simulink model "dynamik_3"  (R2016b)
settings: Solver=ode45  StartTime=0.0  StopTime=80  RelTol=1e-3
values from neighbouring files (symbols this model uses):
  A = 0.05    [Test_m1_init.m]
  a_acc = 1    [Test_m1_init.m]    (also in Test_m2_init.m = 5.5)
  a_de = 1    [Test_m1_init.m]    (also in Test_m2_init.m = 5.5)
  d_2 = 0.15    [Test_m1_init.m]
  dot_phi_soll = 1    [Test_m2_init.m]
  I_R = Mass*(0.5*L)^2    (= 0.08)    [Test_m1_init.m]    (also in Test_m2_init.m)
  L = 0.4    [Test_m1_init.m]    (also in Test_m2_init.m)
  l = 0.2    [Test_m1_init.m]    (also in Test_m2_init.m)
  m = 0.5    [Test_m1_init.m]    (also in Test_m2_init.m)
  Mass = 2    [Test_m1_init.m]    (also in Test_m2_init.m)
libraries: simulink x2
settings Model: Creator=Alexa  LastModifiedBy=Alexa

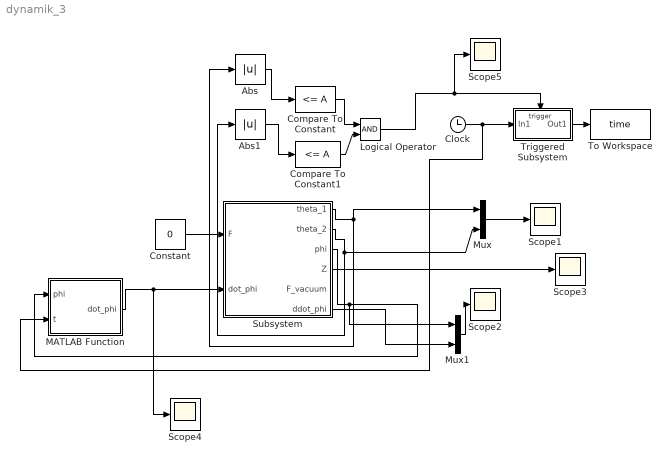
== system dynamik_3 ==
  Abs : Abs
  Abs1 : Abs
  Clock : Clock
  Compare To Constant : simulink/Logic and Bit Operations/Compare To Constant  relop=<=  const=A  OutDataTypeStr=boolean
  Compare To Constant1 : simulink/Logic and Bit Operations/Compare To Constant  relop=<=  const=A  OutDataTypeStr=boolean
  Constant : Constant  Value=0
  Logical Operator : Logic  AllPortsSameDT=off  OutDataTypeStr=boolean
  MATLAB Function : MATLAB Function  TreatAsAtomicUnit=on
  Mux : Mux  Inputs=2
  Mux1 : Mux  Inputs=2
  Scope{1..5} (5 alike) : Scope
  Subsystem : Subsystem
  To Workspace : ToWorkspace  VariableName=time  SaveFormat=Timeseries  SampleTime=-1
  Triggered Subsystem : Subsystem  TreatAsAtomicUnit=on
  wires:
  Subsystem/2(theta_2) -> Abs1/1, Mux/2
  Subsystem/1(theta_1) -> Abs/1, Mux/1
  Constant/1 -> Subsystem/1(F)
  Subsystem/3(phi) -> MATLAB Function/1(phi), Mux1/1
  Subsystem/4(Z) -> Scope3/1
  Compare To Constant/1 -> Logical Operator/1
  Compare To Constant1/1 -> Logical Operator/2
  Logical Operator/1 -> Scope5/1, Triggered Subsystem/Trigger
  Triggered Subsystem/1(Out1) -> To Workspace/1
  MATLAB Function/1(dot_phi) -> Subsystem/2(dot_phi), Scope4/1
  Subsystem/6(ddot_phi) -> Mux1/2
  Mux1/1 -> Scope2/1
  Clock/1 -> MATLAB Function/2(t), Triggered Subsystem/1(In1)
  Mux/1 -> Scope1/1
  Abs/1 -> Compare To Constant/1
  Abs1/1 -> Compare To Constant1/1

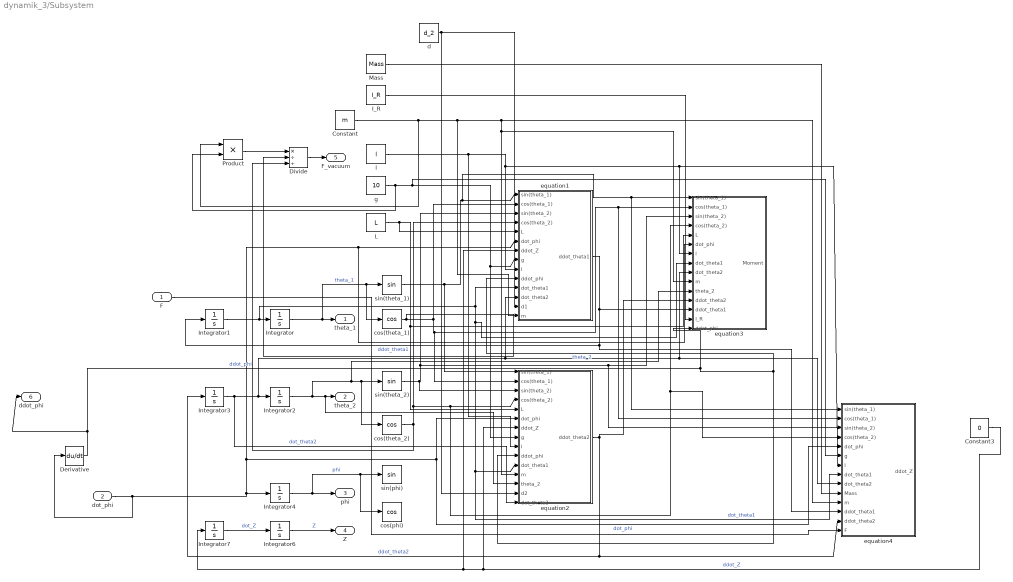
== system dynamik_3/Subsystem ==
  F : Inport
  dot_phi : Inport  Port=2
  Constant : Constant  Value=m
  Constant3 : Constant  Value=0
  Derivative : Derivative
  Divide : Product  Inputs=*//
  I_R : Constant  Value=I_R
  Integrator{,1..4,6..7} (7 alike) : Integrator
  L : Constant  Value=L
  Mass : Constant  Value=Mass
  Product : Product
  cos(phi) : Trigonometry  Operator=cos
  cos(theta_1) : Trigonometry  Operator=cos
  cos(theta_2) : Trigonometry  Operator=cos
  d : Constant  Value=d_2
  equation1 : Subsystem
  equation2 : Subsystem
  equation3 : Subsystem
  equation4 : Subsystem
  g : Constant  Value=10
  l : Constant  Value=l
  sin(phi) : Trigonometry
  sin(theta_1) : Trigonometry
  sin(theta_2) : Trigonometry
  theta_1 : Outport
  theta_2 : Outport  Port=2
  phi : Outport  Port=3
  Z : Outport  Port=4
  F_vacuum : Outport  Port=5
  ddot_phi : Outport  Port=6
  wires:
  Integrator/1 -> cos(theta_1)/1, sin(theta_1)/1, theta_1/1  "theta_1"
  Integrator1/1 -> equation1/11(dot_theta1), equation3/8(dot_theta1), equation4/8(dot_theta1), equation2/11(dot_theta1), Integrator/1  "dot_theta1"
  Integrator2/1 -> equation3/11(theta_2), cos(theta_2)/1, sin(theta_2)/1, equation2/13(theta_2), theta_2/1  "theta_2"
  Integrator3/1 -> equation2/15(dot_theta2), equation4/9(dot_theta2), equation3/9(dot_theta2), equation1/12(dot_theta2), Integrator2/1  "dot_theta2"
  Integrator4/1 -> cos(phi)/1, sin(phi)/1, phi/1  "phi"
  Integrator6/1 -> Z/1  "Z"
  Integrator7/1 -> Integrator6/1  "dot_Z"
  equation1/1(ddot_theta1) -> equation3/13(ddot_theta1), equation4/12(ddot_theta1), Integrator1/1  "ddot_theta1"
  equation2/1(ddot_theta2) -> equation3/12(ddot_theta2), equation4/13(ddot_theta2), Integrator3/1  "ddot_theta2"
  Constant3/1 -> equation1/7(ddot_Z), Integrator7/1, equation2/7(ddot_Z)  "ddot_Z"
  sin(theta_1)/1 -> equation2/1(sin(theta_1)), equation4/1(sin(theta_1)), equation3/1(sin(theta_1)), equation1/1(sin(theta_1))
  cos(theta_1)/1 -> Divide/2, equation2/2(cos(theta_1)), equation4/2(cos(theta_1)), equation3/2(cos(theta_1)), equation1/2(cos(theta_1))
  sin(theta_2)/1 -> equation2/3(sin(theta_2)), equation4/3(sin(theta_2)), equation3/3(sin(theta_2)), equation1/3(sin(theta_2))
  cos(theta_2)/1 -> Divide/3, equation4/4(cos(theta_2)), equation3/4(cos(theta_2)), equation2/4(cos(theta_2)), equation1/4(cos(theta_2))
  L/1 -> equation2/5(L), equation3/5(L), equation1/5(L)
  g/1 -> Product/2, equation4/6(g), equation2/8(g), equation1/8(g)
  l/1 -> equation2/9(l), equation4/7(l), equation3/7(l), equation1/9(l)
  Constant/1 -> Product/1, equation1/14(m), equation4/11(m), equation2/12(m), equation3/10(m)
  I_R/1 -> equation3/14(I_R)
  Mass/1 -> equation4/10(Mass)
  Product/1 -> Divide/1
  Divide/1 -> F_vacuum/1
  d/1 -> equation1/13(d1), equation2/14(d2)
  F/1 -> equation4/14(F)
  Derivative/1 -> ddot_phi/1, equation3/15("ddot_phi "), equation1/10(ddot_phi), equation2/10(ddot_phi)  "ddot_phi"
  dot_phi/1 -> Derivative/1, equation2/6(dot_phi), equation4/5(dot_phi), equation3/6(dot_phi), equation1/6(dot_phi), Integrator4/1  "dot_phi"

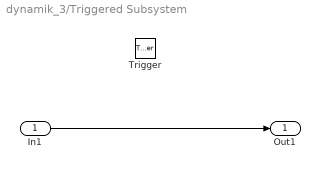
== system dynamik_3/Triggered Subsystem ==
  In1 : Inport
  Trigger : TriggerPort  VariantControl=Variant
  Out1 : Outport
  wires:
  In1/1 -> Out1/1

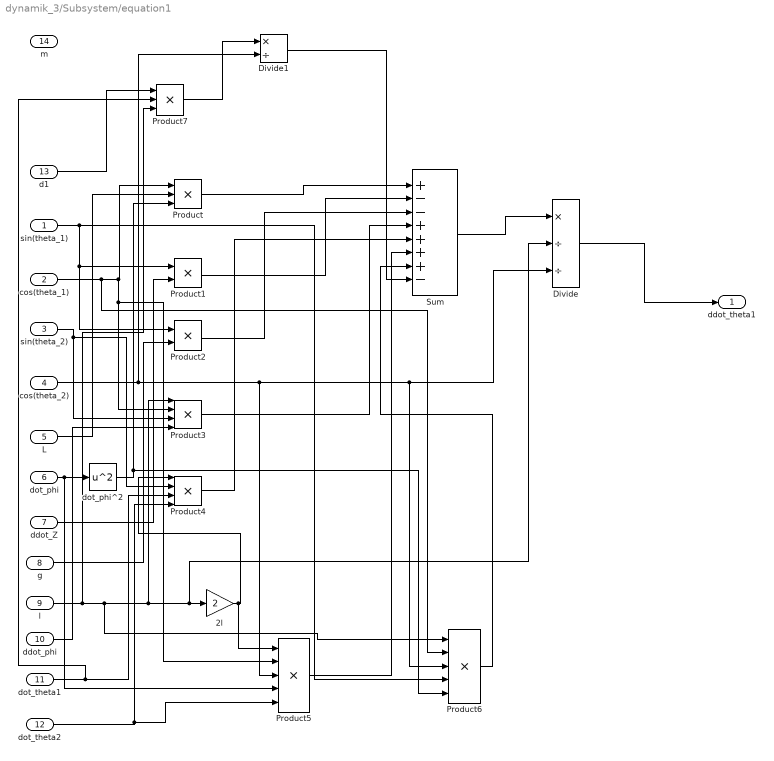
== system dynamik_3/Subsystem/equation1 ==
  sin(theta_1) : Inport
  cos(theta_1) : Inport  Port=2
  sin(theta_2) : Inport  Port=3
  cos(theta_2) : Inport  Port=4
  L : Inport  Port=5
  dot_phi : Inport  Port=6
  ddot_Z : Inport  Port=7
  g : Inport  Port=8
  l : Inport  Port=9
  ddot_phi : Inport  Port=10
  dot_theta1 : Inport  Port=11
  dot_theta2 : Inport  Port=12
  d1 : Inport  Port=13
  m : Inport  Port=14
  2l : Gain  Gain=2
  Divide : Product  Inputs=*//
  Divide1 : Product  Inputs=*/
  Product : Product  Inputs=3
  Product1 : Product
  Product2 : Product
  Product3 : Product  Inputs=4
  Product4 : Product  Inputs=4
  Product5 : Product  Inputs=5
  Product6 : Product  Inputs=5
  Product7 : Product  Inputs=3
  Sum : Sum  Inputs=+--++++-
  dot_phi^2 : Math  Operator=square  SaturateOnIntegerOverflow=on
  ddot_theta1 : Outport
  wires:
  dot_phi/1 -> Product5/4, dot_phi^2/1
  cos(theta_1)/1 -> Product6/2, Product5/2, Product3/2, Product/1
  L/1 -> Product/2
  dot_phi^2/1 -> Product6/5, Product/3
  Product/1 -> Sum/1
  sin(theta_1)/1 -> Product6/4, Product2/1, Product1/1
  Product1/1 -> Sum/2
  ddot_Z/1 -> Product1/2
  g/1 -> Product2/2
  Product2/1 -> Sum/3
  l/1 -> Product7/3, Product6/1, Divide/2, 2l/1, Product3/1
  sin(theta_2)/1 -> Product4/2, Product3/3
  Product3/1 -> Sum/4
  ddot_phi/1 -> Product3/4
  2l/1 -> Product5/1, Product4/1
  dot_theta1/1 -> Product7/2, Product4/3
  dot_theta2/1 -> Product5/5, Product4/4
  Product4/1 -> Sum/5
  cos(theta_2)/1 -> Divide1/2, Divide/3, Product6/3, Product5/3
  Product5/1 -> Sum/6
  Sum/1 -> Divide/1
  Product6/1 -> Sum/7
  Divide/1 -> ddot_theta1/1
  d1/1 -> Product7/1
  Product7/1 -> Divide1/1
  Divide1/1 -> Sum/8

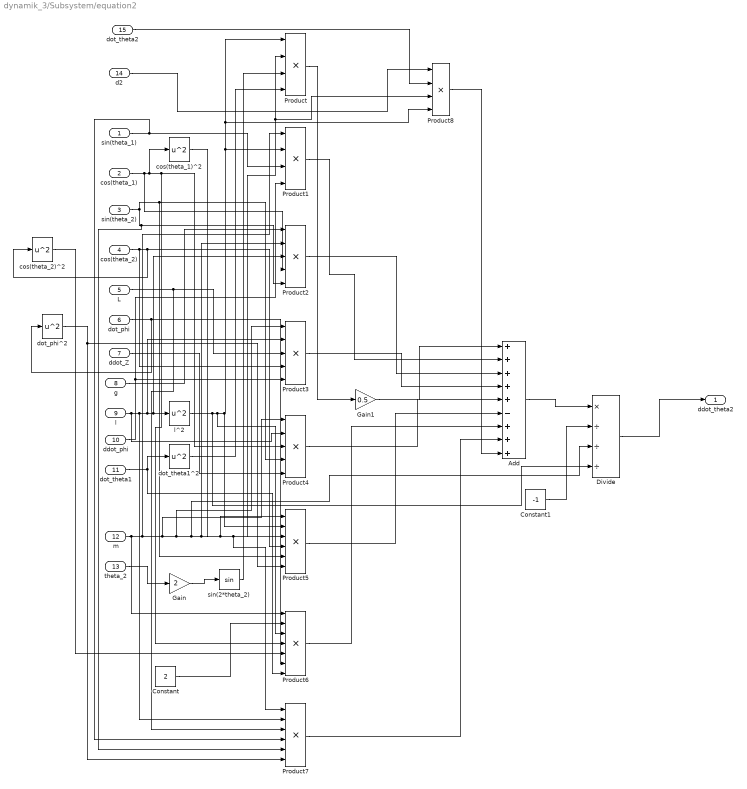
== system dynamik_3/Subsystem/equation2 ==
  sin(theta_1) : Inport
  cos(theta_1) : Inport  Port=2
  sin(theta_2) : Inport  Port=3
  cos(theta_2) : Inport  Port=4
  L : Inport  Port=5
  dot_phi : Inport  Port=6
  ddot_Z : Inport  Port=7
  g : Inport  Port=8
  l : Inport  Port=9
  ddot_phi : Inport  Port=10
  dot_theta1 : Inport  Port=11
  m : Inport  Port=12
  theta_2 : Inport  Port=13
  d2 : Inport  Port=14
  dot_theta2 : Inport  Port=15
  Add : Sum  Inputs=+++++-+++
  Constant : Constant  Value=2
  Constant1 : Constant  Value=-1
  Divide : Product  Inputs=*///
  Gain : Gain  Gain=2
  Gain1 : Gain  Gain=0.5
  Product : Product  Inputs=4
  Product1 : Product  Inputs=4
  Product2 : Product  Inputs=5
  Product3 : Product  Inputs=5
  Product4 : Product  Inputs=5
  Product5 : Product  Inputs=6
  Product6 : Product  Inputs=7
  Product7 : Product  Inputs=6
  Product8 : Product  Inputs=4
  cos(theta_1)^2 : Math  Operator=square  SaturateOnIntegerOverflow=on
  cos(theta_2)^2 : Math  Operator=square  SaturateOnIntegerOverflow=on
  dot_phi^2 : Math  Operator=square  SaturateOnIntegerOverflow=on
  dot_theta1^2 : Math  Operator=square  SaturateOnIntegerOverflow=on
  l^2 : Math  Operator=square  SaturateOnIntegerOverflow=on
  sin(2*theta_2) : Trigonometry
  ddot_theta2 : Outport
  wires:
  l/1 -> Product4/2, Product7/2, Product3/2, Product2/3, l^2/1
  l^2/1 -> Divide/4, Product6/3, Product5/2, Product8/4, Product/1, Product1/2
  m/1 -> Product6/1, Product1/1, Product4/1, Product3/1, Divide/3, Product2/2, Product5/1, Product8/3, Product/2
  theta_2/1 -> Gain/1
  Gain/1 -> sin(2*theta_2)/1
  sin(2*theta_2)/1 -> Product/3
  dot_theta1/1 -> Product6/7, dot_theta1^2/1
  dot_theta1^2/1 -> Product/4
  Product/1 -> Gain1/1
  Gain1/1 -> Add/1
  sin(theta_1)/1 -> Product7/4, Product1/3
  ddot_phi/1 -> Product1/4, Product3/5
  Product1/1 -> Add/2
  g/1 -> Product2/1
  cos(theta_1)/1 -> cos(theta_1)^2/1, Product6/4, Product4/3, Product2/4
  sin(theta_2)/1 -> Product7/5, Product2/5, Product5/5, Product4/4
  Product2/1 -> Add/3
  L/1 -> Product7/3, Product3/3
  cos(theta_2)/1 -> cos(theta_2)^2/1, Product5/4, Product3/4
  Product3/1 -> Add/4
  ddot_Z/1 -> Product4/5
  Product4/1 -> Add/5
  cos(theta_1)^2/1 -> Product7/1, Product5/3
  dot_phi/1 -> Product6/6, dot_phi^2/1
  dot_phi^2/1 -> Product7/6, Product5/6
  Product5/1 -> Add/6
  Constant/1 -> Product6/2
  cos(theta_2)^2/1 -> Product6/5
  Product6/1 -> Add/7
  Product7/1 -> Add/8
  Add/1 -> Divide/1
  Constant1/1 -> Divide/2
  Divide/1 -> ddot_theta2/1
  d2/1 -> Product8/1
  dot_theta2/1 -> Product8/2
  Product8/1 -> Add/9

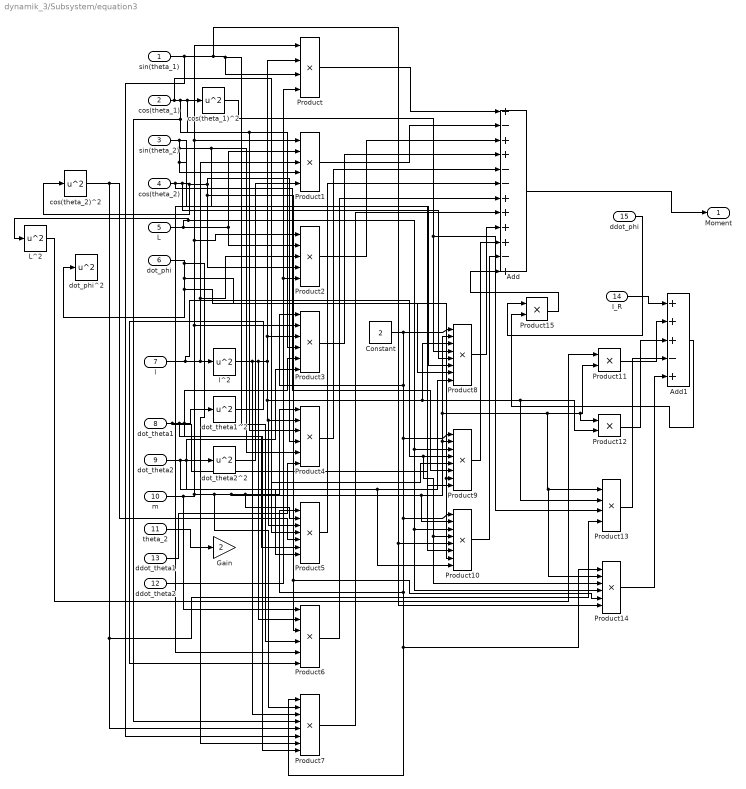
== system dynamik_3/Subsystem/equation3 ==
  sin(theta_1) : Inport
  cos(theta_1) : Inport  Port=2
  sin(theta_2) : Inport  Port=3
  cos(theta_2) : Inport  Port=4
  L : Inport  Port=5
  dot_phi : Inport  Port=6
  l : Inport  Port=7
  dot_theta1 : Inport  Port=8
  dot_theta2 : Inport  Port=9
  m : Inport  Port=10
  theta_2 : Inport  Port=11
  ddot_theta2 : Inport  Port=12
  ddot_theta1 : Inport  Port=13
  I_R : Inport  Port=14
  "ddot_phi " : Inport  Port=15
  Add : Sum  Inputs=+-++--++++-+
  Add1 : Sum  Inputs=+++-+
  Constant : Constant  Value=2
  Gain : Gain  Gain=2
  L^2 : Math  Operator=square  SaturateOnIntegerOverflow=on
  Product : Product  Inputs=4
  Product1 : Product  Inputs=5
  Product{7..10} (4 alike) : Product  Inputs=8
  Product11 : Product
  Product12 : Product
  Product13 : Product  Inputs=4
  Product{3..4,6,14} (4 alike) : Product  Inputs=6
  Product15 : Product
  Product2 : Product  Inputs=5
  Product5 : Product  Inputs=7
  cos(theta_1)^2 : Math  Operator=square  SaturateOnIntegerOverflow=on
  cos(theta_2)^2 : Math  Operator=square  SaturateOnIntegerOverflow=on
  dot_phi^2 : Math  Operator=square  SaturateOnIntegerOverflow=on
  dot_theta1^2 : Math  Operator=square  SaturateOnIntegerOverflow=on
  dot_theta2^2 : Math  Operator=square  SaturateOnIntegerOverflow=on
  l^2 : Math  Operator=square  SaturateOnIntegerOverflow=on
  "Moment " : Outport
  wires:
  l/1 -> Product14/3, Product10/4, Product9/4, Product2/3, Product1/3, l^2/1
  theta_2/1 -> Gain/1
  dot_theta1/1 -> Product9/8, Product7/8, Product5/6, Product3/5, dot_theta1^2/1
  cos(theta_1)/1 -> Product9/5, Product7/4, Product5/4, Product4/3, Product3/4, cos(theta_1)^2/1
  cos(theta_2)/1 -> Product9/6, Product8/5, Product4/4, Product14/5, Product6/3, Product2/4, cos(theta_2)^2/1
  dot_phi/1 -> Product7/7, Product8/7, Product10/7, Product9/7, dot_phi^2/1
  m/1 -> Product6/1, Product7/2, Product10/2, Product9/2, Product14/2, Product13/1, Product12/1, Product11/2, Product8/2, Product5/2, Product4/1, Product3/2, Product2/1, Product1/1, Product/1
  sin(theta_1)/1 -> Product7/6, Product14/6, Product10/5, Product6/4, Product/3
  ddot_theta2/1 -> Product2/5, Product/4
  Product/1 -> Add/1
  L/1 -> L^2/1, Product14/4, Product10/3, Product9/3, Product2/2, Product1/2
  sin(theta_2)/1 -> Product10/6, Product6/5, Product4/5, Product8/6, Product1/4
  dot_theta2^2/1 -> Product1/5
  Product1/1 -> Add/2
  Product2/1 -> Add/3
  Constant/1 -> Product8/1, Product9/1, Product10/1, Product14/1, Product7/1, Product5/1, Product3/1
  Product3/1 -> Add/4
  ddot_theta1/1 -> Product4/6
  Product4/1 -> Add/5
  cos(theta_2)^2/1 -> Product13/4, Product7/5, Product5/5
  Product5/1 -> Add/6
  dot_theta1^2/1 -> Product6/6
  Product6/1 -> Add/7
  Product7/1 -> Add/8
  cos(theta_1)^2/1 -> Product13/3, Product8/4
  Product8/1 -> Add/9
  Product9/1 -> Add/10
  dot_theta2/1 -> Product10/8, Product8/8, Product5/7, Product3/6, dot_theta2^2/1
  Product10/1 -> Add/11
  I_R/1 -> Add1/1
  Product11/1 -> Add1/2
  L^2/1 -> Product11/1
  l^2/1 -> Product7/3, Product6/2, Product13/2, Product12/2, Product8/3, Product5/3, Product4/2, Product3/3, Product/2
  Product12/1 -> Add1/3
  Product13/1 -> Add1/4
  Product14/1 -> Add1/5
  Add1/1 -> Product15/2
  "ddot_phi "/1 -> Product15/1
  Product15/1 -> Add/12
  Add/1 -> "Moment "/1

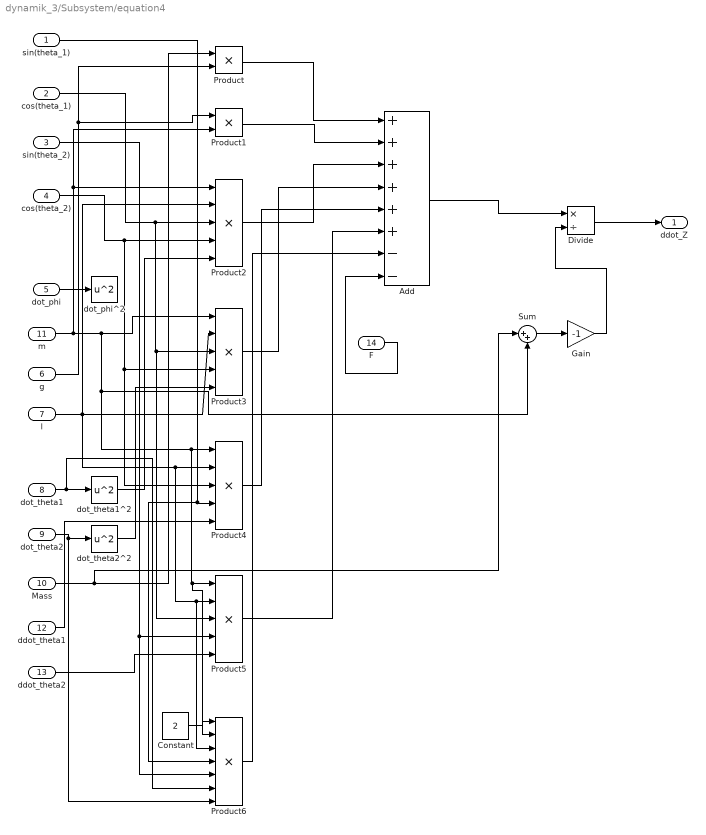
== system dynamik_3/Subsystem/equation4 ==
  sin(theta_1) : Inport
  cos(theta_1) : Inport  Port=2
  sin(theta_2) : Inport  Port=3
  cos(theta_2) : Inport  Port=4
  dot_phi : Inport  Port=5
  g : Inport  Port=6
  l : Inport  Port=7
  dot_theta1 : Inport  Port=8
  dot_theta2 : Inport  Port=9
  Mass : Inport  Port=10
  m : Inport  Port=11
  ddot_theta1 : Inport  Port=12
  ddot_theta2 : Inport  Port=13
  F : Inport  Port=14
  Add : Sum  Inputs=++++++--
  Constant : Constant  Value=2
  Divide : Product  Inputs=*/
  Gain : Gain  Gain=-1
  Product : Product
  Product1 : Product
  Product{2..5} (4 alike) : Product  Inputs=5
  Product6 : Product  Inputs=7
  Sum : Sum  Inputs=|++
  dot_phi^2 : Math  Operator=square  SaturateOnIntegerOverflow=on
  dot_theta1^2 : Math  Operator=square  SaturateOnIntegerOverflow=on
  dot_theta2^2 : Math  Operator=square  SaturateOnIntegerOverflow=on
  ddot_Z : Outport
  wires:
  dot_phi/1 -> dot_phi^2/1
  Mass/1 -> Sum/1, Product/1
  g/1 -> Product1/1, Product/2
  Product/1 -> Add/1
  m/1 -> Sum/2, Product6/2, Product5/1, Product4/1, Product3/1, Product2/1, Product1/2
  Product1/1 -> Add/2
  l/1 -> Product6/3, Product5/2, Product4/2, Product3/2, Product2/2
  cos(theta_1)/1 -> Product5/3, Product3/3, Product2/3
  cos(theta_2)/1 -> Product4/3, Product3/4, Product2/4
  dot_theta1/1 -> Product6/6, dot_theta1^2/1
  dot_theta1^2/1 -> Product2/5
  Product2/1 -> Add/3
  dot_theta2/1 -> Product6/7, dot_theta2^2/1
  dot_theta2^2/1 -> Product3/5
  Product3/1 -> Add/4
  sin(theta_1)/1 -> Product6/4, Product4/4
  ddot_theta1/1 -> Product4/5
  Product4/1 -> Add/5
  sin(theta_2)/1 -> Product6/5, Product5/4
  ddot_theta2/1 -> Product5/5
  Product5/1 -> Add/6
  Constant/1 -> Product6/1
  Product6/1 -> Add/7
  F/1 -> Add/8
  Add/1 -> Divide/1
  Sum/1 -> Gain/1
  Gain/1 -> Divide/2
  Divide/1 -> ddot_Z/1

== matlab function dynamik_3/MATLAB Function ==
  data: phi input; dot_phi output; dot_phi_soll parameter; a_acc parameter; a_de parameter; t input
function dot_phi = fcn(phi,dot_phi_soll,a_acc, a_de,t)
%  if phi<=(0.5*dot_phi_soll^2/a_acc)
%        dot_phi=a_acc*t;
%  elseif phi>(0.5*dot_phi_soll^2/a_acc)&&phi<=(90-0.5*dot_phi_soll^2/a_de)
%        dot_phi=dot_phi_soll;
%  elseif phi<=90&&phi>(90-0.5*dot_phi_soll^2/a_de) 
%        dot_phi=dot_phi_soll-a_de*(t-dot_phi_soll/a_acc-(90-0.5*dot_phi_soll^2/a_acc-0.5*dot_phi_soll^2/a_de)/dot_phi_soll);
%  else
%      dot_phi=0;
%  end

%  if phi<=90
%      dot_phi=dot_phi_soll;
%  else
%      dot_phi=0;
%  end
 m=0.5*dot_phi_soll^2/a_acc;
 q=pi/2-0.5*dot_phi_soll^2/a_de;
 if phi<=m
     dot_phi=min(dot_phi_soll,a_acc*t);
 elseif phi>m&&phi<q
     dot_phi=dot_phi_soll;
 elseif phi>=q&&phi<=pi/2
     dot_phi=max(0,dot_phi_soll-a_de*(t-(q-m)/dot_phi_soll-dot_phi_soll/a_acc));
 else
     dot_phi=0;
 end
end
